simulink model "ModeloPlanta"  (R2015a)
settings: Solver=ode45  StartTime=0.0  StopTime=200  RelTol=1e-3
settings Model: Creator=user  LastModifiedBy=user
settings SolverCC: ZeroCrossControl=DisableAll

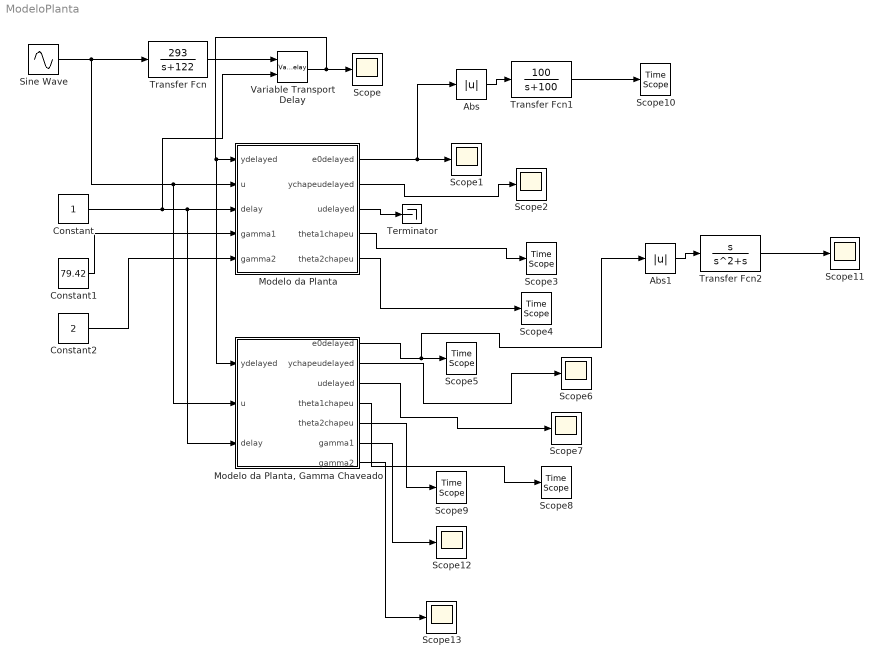
== system ModeloPlanta ==
  Abs : Abs
  Abs1 : Abs
  Constant : Constant
  Constant1 : Constant  Value=79.42
  Constant2 : Constant  Value=2
  Modelo da Planta : Subsystem  Description=First Order Transfer Function Estimation Block
  "Modelo da Planta, Gamma Chaveado" : Subsystem  Description=First Order Transfer Function Estimation Block
  Scope{,1..2,6..7,11..13} (8 alike) : Scope
      Scope1 settings: YMin=-3e-05  YMax=3e-05
      Scope11 settings: YMin=-3.46945e-18  YMax=0.14  SaveName=ScopeData11
      Scope12 settings: YMin=100  YMax=100  SaveName=ScopeData12
      Scope13 settings: YMin=5  SaveName=ScopeData13
      Scope2 settings: YMin=-0.75  YMax=0.75  SaveName=ScopeData2
      Scope6 settings: YMin=-0.35  YMax=0.3  SaveName=ScopeData6
      Scope7 settings: YMin=-1  YMax=1  SaveName=ScopeData7
  Scope{3..5,8..10} (6 alike) : TimeScope
  Sine Wave : Sin  Frequency=10  SampleTime=0
  Terminator : Terminator
  Transfer Fcn : TransferFcn  Numerator=[293]  Denominator=[1 122]
  Transfer Fcn1 : TransferFcn  Numerator=[100]  Denominator=[1 100]
  Transfer Fcn2 : TransferFcn  Numerator=[1 0]  Denominator=[1 1 0]
  Variable Transport Delay : VariableTransportDelay  VariableDelayType=Variable transport delay  MaximumDelay=10  MaximumPoints=4096
  wires:
  Sine Wave/1 -> "Modelo da Planta, Gamma Chaveado"/2(u), Modelo da Planta/2(u), Transfer Fcn/1
  Modelo da Planta/3(udelayed) -> Terminator/1
  Modelo da Planta/4(theta1chapeu) -> Scope3/1
  Modelo da Planta/1(e0delayed) -> Abs/1, Scope1/1
  Modelo da Planta/2(ychapeudelayed) -> Scope2/1
  Modelo da Planta/5(theta2chapeu) -> Scope4/1
  Constant/1 -> Variable Transport Delay/2, "Modelo da Planta, Gamma Chaveado"/3(delay), Modelo da Planta/3(delay)
  Constant1/1 -> Modelo da Planta/4(gamma1)
  Constant2/1 -> Modelo da Planta/5(gamma2)
  Transfer Fcn/1 -> Variable Transport Delay/1
  Variable Transport Delay/1 -> "Modelo da Planta, Gamma Chaveado"/1(ydelayed), Modelo da Planta/1(ydelayed), Scope/1
  "Modelo da Planta, Gamma Chaveado"/2(ychapeudelayed) -> Scope6/1
  "Modelo da Planta, Gamma Chaveado"/3(udelayed) -> Scope7/1
  "Modelo da Planta, Gamma Chaveado"/4(theta1chapeu) -> Scope8/1
  "Modelo da Planta, Gamma Chaveado"/5(theta2chapeu) -> Scope9/1
  Transfer Fcn1/1 -> Scope10/1
  Abs/1 -> Transfer Fcn1/1
  "Modelo da Planta, Gamma Chaveado"/1(e0delayed) -> Abs1/1, Scope5/1
  Transfer Fcn2/1 -> Scope11/1
  Abs1/1 -> Transfer Fcn2/1
  "Modelo da Planta, Gamma Chaveado"/6(gamma1) -> Scope12/1
  "Modelo da Planta, Gamma Chaveado"/7(gamma2) -> Scope13/1

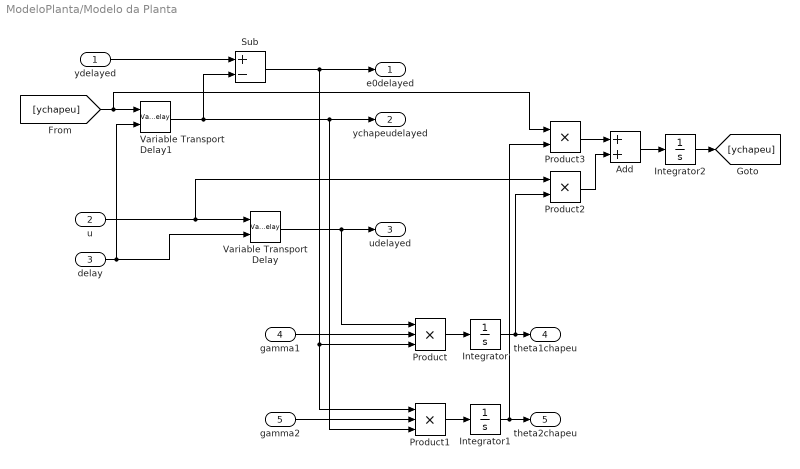
== system ModeloPlanta/Modelo da Planta ==
  ydelayed : Inport
  u : Inport  Port=2
  delay : Inport  Port=3
  gamma1 : Inport  Port=4
  gamma2 : Inport  Port=5
  Add : Sum
  Integrator : Integrator
  Integrator1 : Integrator
  Integrator2 : Integrator
  Product : Product  Inputs=3
  Product1 : Product  Inputs=3
  Product2 : Product
  Product3 : Product
  Sub : Sum  Inputs=+-
  Variable Transport Delay : VariableTransportDelay  VariableDelayType=Variable transport delay  MaximumDelay=10
  Variable Transport Delay1 : VariableTransportDelay  VariableDelayType=Variable transport delay  MaximumDelay=10
  e0delayed : Outport
  ychapeudelayed : Outport  Port=2
  udelayed : Outport  Port=3
  theta1chapeu : Outport  Port=4
  theta2chapeu : Outport  Port=5
  wires:
  ydelayed/1 -> Sub/1
  Sub/1 -> Product1/1, Product/3, e0delayed/1
  delay/1 -> Variable Transport Delay1/2, Variable Transport Delay/2
  u/1 -> Product2/1, Variable Transport Delay/1
  Variable Transport Delay/1 -> Product/1, udelayed/1
  gamma1/1 -> Product/2
  Product/1 -> Integrator/1
  Integrator/1 -> Product2/2, theta1chapeu/1
  gamma2/1 -> Product1/2
  [ychapeu] -> Product3/1, Variable Transport Delay1/1
  Variable Transport Delay1/1 -> Product1/3, ychapeudelayed/1, Sub/2
  Product1/1 -> Integrator1/1
  Integrator1/1 -> Product3/2, theta2chapeu/1
  Product3/1 -> Add/1
  Product2/1 -> Add/2
  Add/1 -> Integrator2/1
  Integrator2/1 -> [ychapeu]

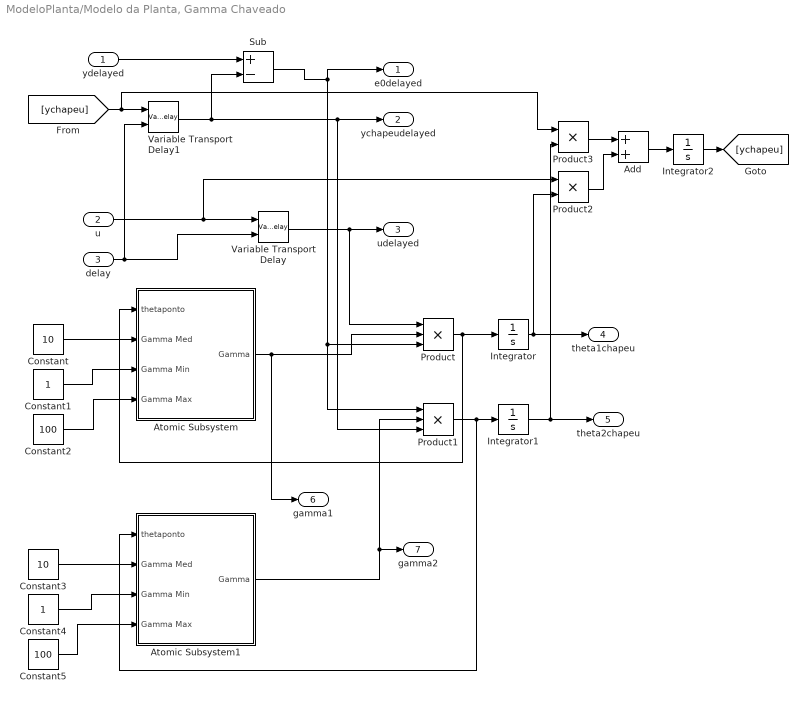
== system ModeloPlanta/Modelo da Planta, Gamma Chaveado ==
  ydelayed : Inport
  u : Inport  Port=2
  delay : Inport  Port=3
  Add : Sum
  Atomic Subsystem : Subsystem  TreatAsAtomicUnit=on
  Atomic Subsystem1 : Subsystem  TreatAsAtomicUnit=on
  Constant : Constant  Value=10
  Constant1 : Constant
  Constant2 : Constant  Value=100
  Constant3 : Constant  Value=10
  Constant4 : Constant
  Constant5 : Constant  Value=100
  Integrator : Integrator
  Integrator1 : Integrator
  Integrator2 : Integrator
  Product : Product  Inputs=3
  Product1 : Product  Inputs=3
  Product2 : Product
  Product3 : Product
  Sub : Sum  Inputs=+-
  Variable Transport Delay : VariableTransportDelay  VariableDelayType=Variable transport delay  MaximumDelay=10
  Variable Transport Delay1 : VariableTransportDelay  VariableDelayType=Variable transport delay  MaximumDelay=10
  e0delayed : Outport
  ychapeudelayed : Outport  Port=2
  udelayed : Outport  Port=3
  theta1chapeu : Outport  Port=4
  theta2chapeu : Outport  Port=5
  gamma1 : Outport  Port=6
  gamma2 : Outport  Port=7
  wires:
  ydelayed/1 -> Sub/1
  Sub/1 -> Product1/1, Product/3, e0delayed/1
  delay/1 -> Variable Transport Delay1/2, Variable Transport Delay/2
  u/1 -> Product2/1, Variable Transport Delay/1
  Variable Transport Delay/1 -> Product/1, udelayed/1
  Atomic Subsystem/1(Gamma) -> gamma1/1, Product/2
  Product/1 -> Atomic Subsystem/1(thetaponto), Integrator/1
  Integrator/1 -> Product2/2, theta1chapeu/1
  Atomic Subsystem1/1(Gamma) -> gamma2/1, Product1/2
  [ychapeu] -> Product3/1, Variable Transport Delay1/1
  Variable Transport Delay1/1 -> Product1/3, ychapeudelayed/1, Sub/2
  Product1/1 -> Atomic Subsystem1/1(thetaponto), Integrator1/1
  Integrator1/1 -> Product3/2, theta2chapeu/1
  Product3/1 -> Add/1
  Product2/1 -> Add/2
  Add/1 -> Integrator2/1
  Integrator2/1 -> [ychapeu]
  Constant/1 -> Atomic Subsystem/2(Gamma Med)
  Constant1/1 -> Atomic Subsystem/3(Gamma Min)
  Constant2/1 -> Atomic Subsystem/4(Gamma Max)
  Constant3/1 -> Atomic Subsystem1/2(Gamma Med)
  Constant4/1 -> Atomic Subsystem1/3(Gamma Min)
  Constant5/1 -> Atomic Subsystem1/4(Gamma Max)

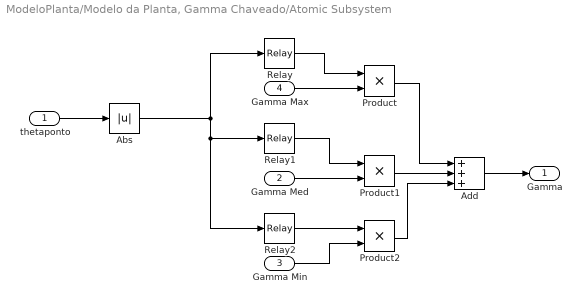
== system ModeloPlanta/Modelo da Planta, Gamma Chaveado/Atomic Subsystem ==
  thetaponto : Inport
  Gamma Med : Inport  Port=2
  Gamma Min : Inport  Port=3
  Gamma Max : Inport  Port=4
  Abs : Abs
  Add : Sum  Inputs=+++
  Product : Product
  Product1 : Product
  Product2 : Product
  Relay : Relay  OnSwitchValue=10  OffSwitchValue=10  OnOutputValue=0  OffOutputValue=1
  Relay1 : Relay  OnSwitchValue=100  OffSwitchValue=100  OnOutputValue=0  OffOutputValue=1
  Relay2 : Relay  OnSwitchValue=1000  OffSwitchValue=1000  OnOutputValue=0  OffOutputValue=1
  Gamma : Outport
  wires:
  thetaponto/1 -> Abs/1
  Gamma Max/1 -> Product/2
  Relay/1 -> Product/1
  Gamma Med/1 -> Product1/2
  Relay1/1 -> Product1/1
  Relay2/1 -> Product2/1
  Gamma Min/1 -> Product2/2
  Product/1 -> Add/1
  Product1/1 -> Add/2
  Product2/1 -> Add/3
  Add/1 -> Gamma/1
  Abs/1 -> Relay2/1, Relay1/1, Relay/1

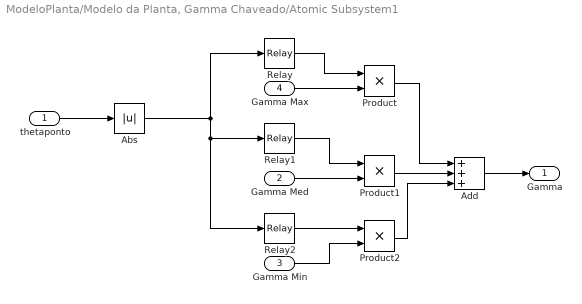
== system ModeloPlanta/Modelo da Planta, Gamma Chaveado/Atomic Subsystem1 ==
  thetaponto : Inport
  Gamma Med : Inport  Port=2
  Gamma Min : Inport  Port=3
  Gamma Max : Inport  Port=4
  Abs : Abs
  Add : Sum  Inputs=+++
  Product : Product
  Product1 : Product
  Product2 : Product
  Relay : Relay  OnSwitchValue=10  OffSwitchValue=10  OnOutputValue=0  OffOutputValue=1
  Relay1 : Relay  OnSwitchValue=100  OffSwitchValue=100  OnOutputValue=0  OffOutputValue=1
  Relay2 : Relay  OnSwitchValue=1000  OffSwitchValue=1000  OnOutputValue=0  OffOutputValue=1
  Gamma : Outport
  wires:
  thetaponto/1 -> Abs/1
  Gamma Max/1 -> Product/2
  Relay/1 -> Product/1
  Gamma Med/1 -> Product1/2
  Relay1/1 -> Product1/1
  Relay2/1 -> Product2/1
  Gamma Min/1 -> Product2/2
  Product/1 -> Add/1
  Product1/1 -> Add/2
  Product2/1 -> Add/3
  Add/1 -> Gamma/1
  Abs/1 -> Relay2/1, Relay1/1, Relay/1
